simulink model "DSB_FC"  (R2020b)
settings: Solver=VariableStepAuto  StartTime=0.0  StopTime=10.0  RelTol=1e-3
libraries: dsparch4 x1
settings Model: Creator=taone  LastModifiedBy=htn
settings SFSimCC: CustomCodeUndefinedFunction=UseInterfaceOnly

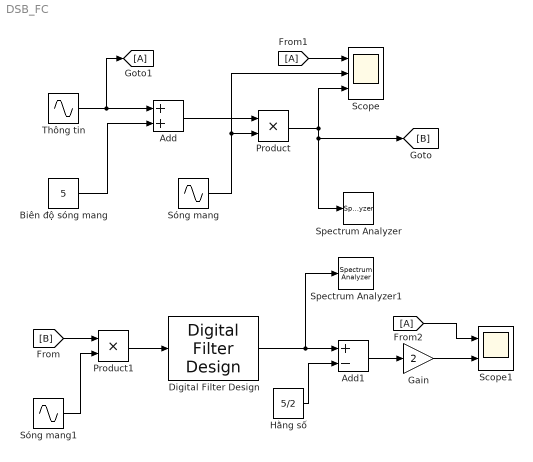
== system DSB_FC ==
  Add : Sum
  Add1 : Sum  Inputs=+-
  Biên độ sóng mang : Constant  Value=5
  Digital Filter Design : dsparch4/Digital Filter Design  mwdsp_browser_bugfix_var=off
  Gain : Gain  Gain=2
  Hằng số : Constant  Value=5/2
  Product : Product
  Product1 : Product
  Scope : Scope  NumInputPorts=3
  Scope1 : Scope  NumInputPorts=2
  Spectrum Analyzer : SpectrumAnalyzer
  Spectrum Analyzer1 : SpectrumAnalyzer
  Sóng mang : Sin  Frequency=2*pi*5000  SampleTime=1/80000
  Sóng mang1 : Sin  Frequency=2*pi*5000  SampleTime=1/80000
  Thông tin : Sin  Amplitude=2  Frequency=2*pi*500  SampleTime=1/80000
  wires:
  Digital Filter Design/1 -> Spectrum Analyzer1/1, Add1/1
  Thông tin/1 -> [A], Add/1
  Biên độ sóng mang/1 -> Add/2
  Add1/1 -> Gain/1
  Gain/1 -> Scope1/2
  Hằng số/1 -> Add1/2
  [A] -> Scope1/1
  [A] -> Scope/1
  Product/1 -> [B], Spectrum Analyzer/1, Scope/3
  [B] -> Product1/1
  Sóng mang1/1 -> Product1/2
  Product1/1 -> Digital Filter Design/1
  Add/1 -> Product/1
  Sóng mang/1 -> Scope/2, Product/2
